simulink library "IO"  (R2024a)
settings: Solver=VariableStepAuto  StartTime=0.0  StopTime=10.0  RelTol=1e-3
values from neighbouring files (symbols this model uses):
  ADCBits = 12.0    [IO.sldd]
  Vref = 5.0    [IO.sldd]
undefined symbols (not defined in the file or in its folder): Bridge, dt, H, raptor_xcp_function
libraries: Raptor_lib x69, Utilities x20, Cooling x1
(part 1 of 3)
settings Model: Creator=serga  LastModifiedBy=hyuga
settings ConfigComp: CovBoundaryAbsTol=1.0e-5

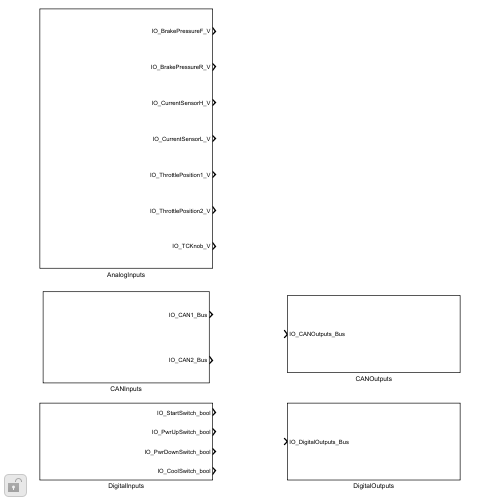
[thumbnail: Simulink's stored preview of the top-level diagram]
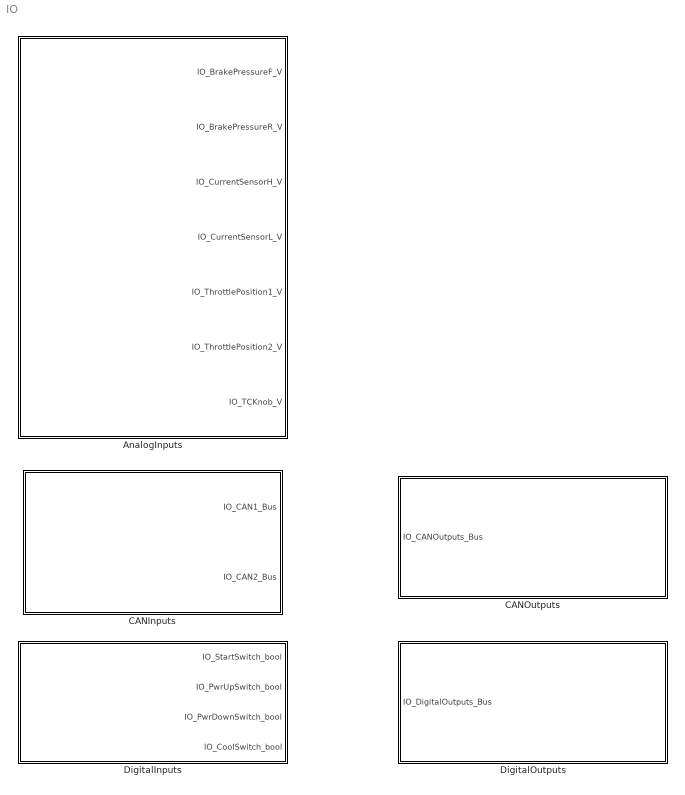
== system IO ==
  AnalogInputs : Subsystem
  CANInputs : Subsystem
  CANOutputs : Subsystem
  DigitalInputs : Subsystem
  DigitalOutputs : Subsystem

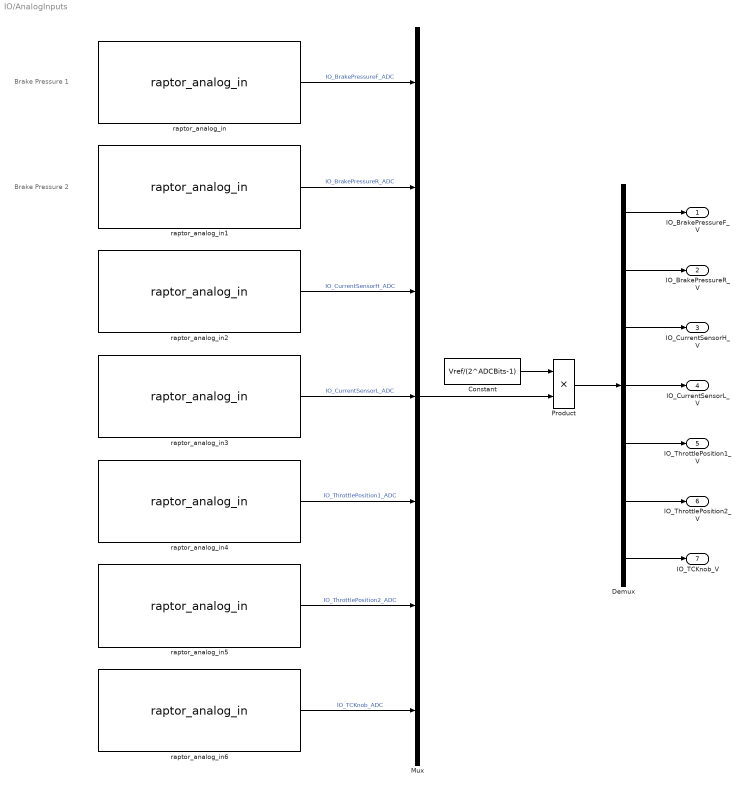
== system IO/AnalogInputs ==
  note: Brake Pressure 2
  note: Brake Pressure 1
  Constant : Constant  Value=Vref/(2^ADCBits-1)
  Demux : Demux  Outputs=7
  Mux : Mux  Inputs=7
  Product : Product
  raptor_analog_in : Raptor_lib/Input & Output/raptor_analog_in  resourceValues=INPUT2|INPUT3|INPUT4|INPUT5|INPUT6|INPUT7|INPUT8|INPUT9|INPUT10|INPUT11|INPUT12|INPUT13|INPUT14|INPUT15|INPUT16|INPUT17|INPUT18|INPUT19|INPUT20|INPUT21|INPUT22|INPUT23|INPUT24|INPUT25|INPUT26|INPUT27|INPUT28|INPUT29|INPUT30|INPUT31|INPUT32|(None)  resource=INPUT4  rangeValues=0 - 5 V  range=0 - 5 V  filterrateValues=[]  filterrate='RAPTOR MASK DEFAULT'  resolutionValues=[]  resolution=[]  pullUDValues=422k PD  pullUD=422k PD
      settings: SourceProductName=Raptor
  raptor_analog_in1 : Raptor_lib/Input & Output/raptor_analog_in  resourceValues=INPUT2|INPUT3|INPUT4|INPUT5|INPUT6|INPUT7|INPUT8|INPUT9|INPUT10|INPUT11|INPUT12|INPUT13|INPUT14|INPUT15|INPUT16|INPUT17|INPUT18|INPUT19|INPUT20|INPUT21|INPUT22|INPUT23|INPUT24|INPUT25|INPUT26|INPUT27|INPUT28|INPUT29|INPUT30|INPUT31|INPUT32|(None)  resource=INPUT12  rangeValues=0 - 5 V  range=0 - 5 V  filterrateValues=[]  filterrate='RAPTOR MASK DEFAULT'  resolutionValues=[]  resolution=[]  pullUDValues=422k PD  pullUD=422k PD
      settings: SourceProductName=Raptor
  raptor_analog_in2 : Raptor_lib/Input & Output/raptor_analog_in  resourceValues=INPUT2|INPUT3|INPUT4|INPUT5|INPUT6|INPUT7|INPUT8|INPUT9|INPUT10|INPUT11|INPUT12|INPUT13|INPUT14|INPUT15|INPUT16|INPUT17|INPUT18|INPUT19|INPUT20|INPUT21|INPUT22|INPUT23|INPUT24|INPUT25|INPUT26|INPUT27|INPUT28|INPUT29|INPUT30|INPUT31|INPUT32|(None)  resource=INPUT13  rangeValues=0 - 5 V  range=0 - 5 V  filterrateValues=[]  filterrate='RAPTOR MASK DEFAULT'  resolutionValues=[]  resolution=[]  pullUDValues=2.15k PU, 31.6k PD  pullUD=2.15k PU, 31.6k PD
      settings: SourceProductName=Raptor
  raptor_analog_in3 : Raptor_lib/Input & Output/raptor_analog_in  resourceValues=INPUT2|INPUT3|INPUT4|INPUT5|INPUT6|INPUT7|INPUT8|INPUT9|INPUT10|INPUT11|INPUT12|INPUT13|INPUT14|INPUT15|INPUT16|INPUT17|INPUT18|INPUT19|INPUT20|INPUT21|INPUT22|INPUT23|INPUT24|INPUT25|INPUT26|INPUT27|INPUT28|INPUT29|INPUT30|INPUT31|INPUT32|(None)  resource=INPUT15  rangeValues=0 - 5 V  range=0 - 5 V  filterrateValues=[]  filterrate='RAPTOR MASK DEFAULT'  resolutionValues=[]  resolution=[]  pullUDValues=2.15k PU, 31.6k PD  pullUD=2.15k PU, 31.6k PD
      settings: SourceProductName=Raptor
  raptor_analog_in4 : Raptor_lib/Input & Output/raptor_analog_in  resourceValues=INPUT2|INPUT3|INPUT4|INPUT5|INPUT6|INPUT7|INPUT8|INPUT9|INPUT10|INPUT11|INPUT12|INPUT13|INPUT14|INPUT15|INPUT16|INPUT17|INPUT18|INPUT19|INPUT20|INPUT21|INPUT22|INPUT23|INPUT24|INPUT25|INPUT26|INPUT27|INPUT28|INPUT29|INPUT30|INPUT31|INPUT32|(None)  resource=INPUT23  rangeValues=0 - 5 V  range=0 - 5 V  filterrateValues=[]  filterrate='RAPTOR MASK DEFAULT'  resolutionValues=[]  resolution=[]  pullUDValues=56.7k PD  pullUD=56.7k PD
      settings: SourceProductName=Raptor
  raptor_analog_in5 : Raptor_lib/Input & Output/raptor_analog_in  resourceValues=INPUT2|INPUT3|INPUT4|INPUT5|INPUT6|INPUT7|INPUT8|INPUT9|INPUT10|INPUT11|INPUT12|INPUT13|INPUT14|INPUT15|INPUT16|INPUT17|INPUT18|INPUT19|INPUT20|INPUT21|INPUT22|INPUT23|INPUT24|INPUT25|INPUT26|INPUT27|INPUT28|INPUT29|INPUT30|INPUT31|INPUT32|(None)  resource=INPUT24  rangeValues=0 - 5 V  range=0 - 5 V  filterrateValues=[]  filterrate='RAPTOR MASK DEFAULT'  resolutionValues=[]  resolution=[]  pullUDValues=56.7k PD  pullUD=56.7k PD
      settings: SourceProductName=Raptor
  raptor_analog_in6 : Raptor_lib/Input & Output/raptor_analog_in  resourceValues=INPUT2|INPUT3|INPUT4|INPUT5|INPUT6|INPUT7|INPUT8|INPUT9|INPUT10|INPUT11|INPUT12|INPUT13|INPUT14|INPUT15|INPUT16|INPUT17|INPUT18|INPUT19|INPUT20|INPUT21|INPUT22|INPUT23|INPUT24|INPUT25|INPUT26|INPUT27|INPUT28|INPUT29|INPUT30|INPUT31|INPUT32|(None)  resource=INPUT29  rangeValues=0 - 5 V  range=0 - 5 V  filterrateValues=[]  filterrate='RAPTOR MASK DEFAULT'  resolutionValues=[]  resolution=[]  pullUDValues=215k PD  pullUD=215k PD
      settings: SourceProductName=Raptor
  IO_BrakePressureF_V : Outport
  IO_BrakePressureR_V : Outport  Port=2
  IO_CurrentSensorH_V : Outport  Port=3
  IO_CurrentSensorL_V : Outport  Port=4
  IO_ThrottlePosition1_V : Outport  Port=5
  IO_ThrottlePosition2_V : Outport  Port=6
  IO_TCKnob_V : Outport  Port=7
  wires:
  Demux/7 -> IO_TCKnob_V/1
  Demux/6 -> IO_ThrottlePosition2_V/1
  Demux/5 -> IO_ThrottlePosition1_V/1
  Demux/4 -> IO_CurrentSensorL_V/1
  Demux/3 -> IO_CurrentSensorH_V/1
  Demux/2 -> IO_BrakePressureR_V/1
  Demux/1 -> IO_BrakePressureF_V/1
  raptor_analog_in6/1 -> Mux/7  "IO_TCKnob_ADC"
  raptor_analog_in5/1 -> Mux/6  "IO_ThrottlePosition2_ADC"
  raptor_analog_in4/1 -> Mux/5  "IO_ThrottlePosition1_ADC"
  raptor_analog_in3/1 -> Mux/4  "IO_CurrentSensorL_ADC"
  raptor_analog_in2/1 -> Mux/3  "IO_CurrentSensorH_ADC"
  raptor_analog_in1/1 -> Mux/2  "IO_BrakePressureR_ADC"
  raptor_analog_in/1 -> Mux/1  "IO_BrakePressureF_ADC"
  Product/1 -> Demux/1
  Constant/1 -> Product/1
  Mux/1 -> Product/2

== system IO/CANInputs ==
  CAN1 : Subsystem
  CAN2 : Subsystem
  IO_CAN1_Bus : Outport
  IO_CAN2_Bus : Outport  Port=2
  wires:
  CAN2/1(IO_CAN2_Bus) -> IO_CAN2_Bus/1
  CAN1/1(Out1) -> IO_CAN1_Bus/1

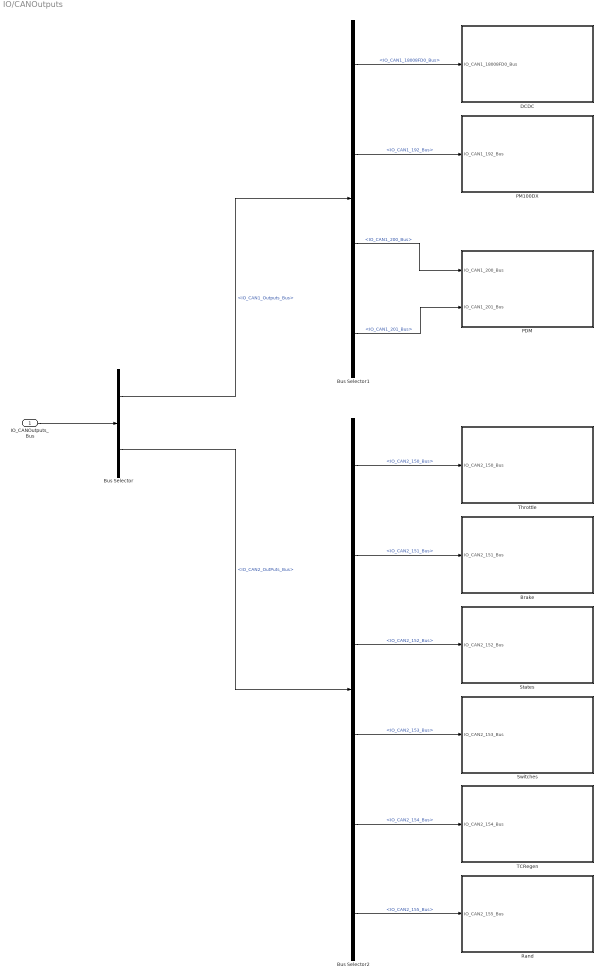
== system IO/CANOutputs ==
  IO_CANOutputs_Bus : Inport
  Brake : Subsystem
  Bus Selector : BusSelector  OutputSignals=IO_CAN1_Outputs_Bus,IO_CAN2_OutPuts_Bus
  Bus Selector1 : BusSelector  OutputSignals=IO_CAN1_18008FD0_Bus,IO_CAN1_192_Bus,IO_CAN1_200_Bus,IO_CAN1_201_Bus
  Bus Selector2 : BusSelector  OutputSignals=IO_CAN2_150_Bus,IO_CAN2_151_Bus,IO_CAN2_152_Bus,IO_CAN2_153_Bus,IO_CAN2_154_Bus,IO_CAN2_155_Bus
  DCDC : Subsystem
  PDM : Subsystem
  PM100DX : Subsystem
  Rand : Subsystem
  States : Subsystem
  Switches : Subsystem
  TCRegen : Subsystem
  Throttle : Subsystem
  wires:
  Bus Selector/2 -> Bus Selector2/1  "<IO_CAN2_OutPuts_Bus>"
  Bus Selector/1 -> Bus Selector1/1  "<IO_CAN1_Outputs_Bus>"
  IO_CANOutputs_Bus/1 -> Bus Selector/1
  Bus Selector1/1 -> DCDC/1(IO_CAN1_18008FD0_Bus)  "<IO_CAN1_18008FD0_Bus>"
  Bus Selector1/2 -> PM100DX/1(IO_CAN1_192_Bus)  "<IO_CAN1_192_Bus>"
  Bus Selector1/3 -> PDM/1(IO_CAN1_200_Bus)  "<IO_CAN1_200_Bus>"
  Bus Selector2/1 -> Throttle/1(IO_CAN2_150_Bus)  "<IO_CAN2_150_Bus>"
  Bus Selector2/2 -> Brake/1(IO_CAN2_151_Bus)  "<IO_CAN2_151_Bus>"
  Bus Selector2/3 -> States/1(IO_CAN2_152_Bus)  "<IO_CAN2_152_Bus>"
  Bus Selector2/4 -> Switches/1(IO_CAN2_153_Bus)  "<IO_CAN2_153_Bus>"
  Bus Selector1/4 -> PDM/2(IO_CAN1_201_Bus)  "<IO_CAN1_201_Bus>"
  Bus Selector2/5 -> TCRegen/1(IO_CAN2_154_Bus)  "<IO_CAN2_154_Bus>"
  Bus Selector2/6 -> Rand/1(IO_CAN2_155_Bus)  "<IO_CAN2_155_Bus>"

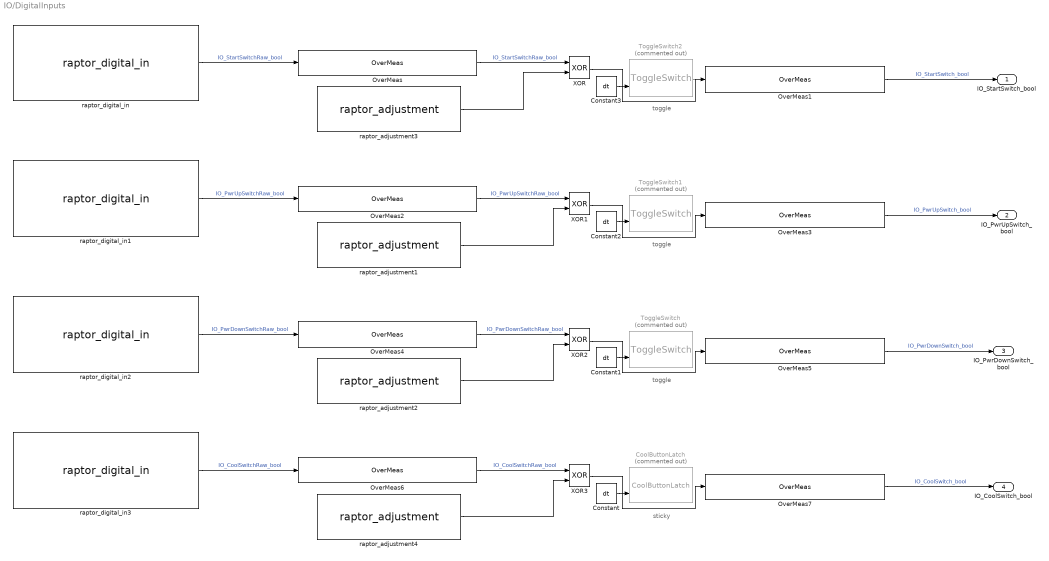
== system IO/DigitalInputs ==
  note: toggle
  note: toggle
  note: sticky
  note: toggle
  Constant{,1..3} (4 alike) : Constant  Value=dt
  CoolButtonLatch : Cooling/CoolButtonLatch  Commented=on  SystemSampleTime=-1  VariantActivationTime=update diagram  EmptyChoice=off  PassThrough=off  PassThroughVariantControl=(default)  EmptyChoiceVariantControl=(default)  AllowFlexibleInterface=on  Latency=0  AutoFrameSizeCalculation=off
  OverMeas : Utilities/OverMeas  sigName='IO_StartSwitchRaw_bool'  minimum=0  maximum=1
  OverMeas1 : Utilities/OverMeas  sigName='IO_StartSwitch_bool'  minimum=0  maximum=1
  OverMeas2 : Utilities/OverMeas  sigName='IO_PwrUpSwitchRaw_bool'  minimum=0  maximum=1
  OverMeas3 : Utilities/OverMeas  sigName='IO_PwrUpSwitch_bool'  minimum=0  maximum=1
  OverMeas4 : Utilities/OverMeas  sigName='IO_PwrDownSwitchRaw_bool'  minimum=0  maximum=1
  OverMeas5 : Utilities/OverMeas  sigName='IO_PwrDownSwitch_bool'  minimum=0  maximum=1
  OverMeas6 : Utilities/OverMeas  sigName='IO_CoolSwitchRaw_bool'  minimum=0  maximum=1
  OverMeas7 : Utilities/OverMeas  sigName='IO_CoolSwitch_bool'  minimum=0  maximum=1
  ToggleSwitch : Utilities/ToggleSwitch  Commented=on  SystemSampleTime=-1  VariantActivationTime=update diagram  EmptyChoice=off  PassThrough=off  PassThroughVariantControl=(default)  EmptyChoiceVariantControl=(default)  AllowFlexibleInterface=on  Latency=0  AutoFrameSizeCalculation=off
  ToggleSwitch1 : Utilities/ToggleSwitch  Commented=on  SystemSampleTime=-1  VariantActivationTime=update diagram  EmptyChoice=off  PassThrough=off  PassThroughVariantControl=(default)  EmptyChoiceVariantControl=(default)  AllowFlexibleInterface=on  Latency=0  AutoFrameSizeCalculation=off
  ToggleSwitch2 : Utilities/ToggleSwitch  Commented=on  SystemSampleTime=-1  VariantActivationTime=update diagram  EmptyChoice=off  PassThrough=off  PassThroughVariantControl=(default)  EmptyChoiceVariantControl=(default)  AllowFlexibleInterface=on  Latency=0  AutoFrameSizeCalculation=off
  XOR{,1..3} (4 alike) : Logic  Operator=XOR  AllPortsSameDT=off  OutDataTypeStr=boolean
  raptor_adjustment1 : Raptor_lib/Data Storage/raptor_adjustment  paramName='IO_PwrUpSwitchPolarity_bool'  nameSource=Parameter  initValue=1  dataType=uint8  storage=Calibration  calDispType=Number  calEnum={'False', 'True'}  calGain=1.0  calOffset=0.0  calMax=inf  calMin=-inf  calFormat='-1'  calUnit=''  calHelp=''  calAccess=1  calFunction=raptor_xcp_function(gcb)  calDispHeaders=off  calColHeaders={'Col1' 'Col2' 'Col3'}  calRowHeaders={'Row1' 'Row2' 'Row3'}
      settings: SourceProductName=Raptor
  raptor_adjustment2 : Raptor_lib/Data Storage/raptor_adjustment  paramName='IO_PwrDownSwitchPolarity_bool'  nameSource=Parameter  initValue=1  dataType=uint8  storage=Calibration  calDispType=Number  calEnum={'False', 'True'}  calGain=1.0  calOffset=0.0  calMax=inf  calMin=-inf  calFormat='-1'  calUnit=''  calHelp=''  calAccess=1  calFunction=raptor_xcp_function(gcb)  calDispHeaders=off  calColHeaders={'Col1' 'Col2' 'Col3'}  calRowHeaders={'Row1' 'Row2' 'Row3'}
      settings: SourceProductName=Raptor
  raptor_adjustment3 : Raptor_lib/Data Storage/raptor_adjustment  paramName='IO_StartSwitchPolarity_bool'  nameSource=Parameter  initValue=0.00  dataType=uint8  storage=Calibration  calDispType=Number  calEnum={'False', 'True'}  calGain=1.0  calOffset=0.0  calMax=inf  calMin=-inf  calFormat='-1'  calUnit=''  calHelp=''  calAccess=1  calFunction=raptor_xcp_function(gcb)  calDispHeaders=off  calColHeaders={'Col1' 'Col2' 'Col3'}  calRowHeaders={'Row1' 'Row2' 'Row3'}
      settings: SourceProductName=Raptor
  raptor_adjustment4 : Raptor_lib/Data Storage/raptor_adjustment  paramName='IO_CoolSwitchPolarity_bool'  nameSource=Parameter  initValue=1  dataType=uint8  storage=Calibration  calDispType=Number  calEnum={'False', 'True'}  calGain=1.0  calOffset=0.0  calMax=inf  calMin=-inf  calFormat='-1'  calUnit=''  calHelp=''  calAccess=1  calFunction=raptor_xcp_function(gcb)  calDispHeaders=off  calColHeaders={'Col1' 'Col2' 'Col3'}  calRowHeaders={'Row1' 'Row2' 'Row3'}
      settings: SourceProductName=Raptor
  raptor_digital_in : Raptor_lib/Input & Output/raptor_digital_in  resourceValues=WAKE_INPUT1|INPUT33|INPUT34|INPUT35|INPUT36|INPUT37|INPUT38|INPUT39|INPUT40|(None)  resource=INPUT35  pullUDValues=1.3k PD  pullUD=1.3k PD  upperThres='RAPTOR MASK DEFAULT'  lowerThres='RAPTOR MASK DEFAULT'
      settings: SourceProductName=Raptor
  raptor_digital_in1 : Raptor_lib/Input & Output/raptor_digital_in  resourceValues=WAKE_INPUT1|INPUT33|INPUT34|INPUT35|INPUT36|INPUT37|INPUT38|INPUT39|INPUT40|(None)  resource=INPUT37  pullUDValues=1.3k PU  pullUD=1.3k PU  upperThres='RAPTOR MASK DEFAULT'  lowerThres='RAPTOR MASK DEFAULT'
      settings: SourceProductName=Raptor
  raptor_digital_in2 : Raptor_lib/Input & Output/raptor_digital_in  resourceValues=WAKE_INPUT1|INPUT33|INPUT34|INPUT35|INPUT36|INPUT37|INPUT38|INPUT39|INPUT40|(None)  resource=INPUT39  pullUDValues=1.3k PU  pullUD=1.3k PU  upperThres='RAPTOR MASK DEFAULT'  lowerThres='RAPTOR MASK DEFAULT'
      settings: SourceProductName=Raptor
  raptor_digital_in3 : Raptor_lib/Input & Output/raptor_digital_in  resourceValues=WAKE_INPUT1|INPUT33|INPUT34|INPUT35|INPUT36|INPUT37|INPUT38|INPUT39|INPUT40|(None)  resource=INPUT40  pullUDValues=1.3k PU  pullUD=1.3k PU  upperThres='RAPTOR MASK DEFAULT'  lowerThres='RAPTOR MASK DEFAULT'
      settings: SourceProductName=Raptor
  IO_StartSwitch_bool : Outport
  IO_PwrUpSwitch_bool : Outport  Port=2
  IO_PwrDownSwitch_bool : Outport  Port=3
  IO_CoolSwitch_bool : Outport  Port=4
  wires:
  ToggleSwitch2/1 -> ?
  XOR/1 -> OverMeas1/1
  Constant3/1 -> ToggleSwitch2/2
  Constant2/1 -> ToggleSwitch1/2
  Constant1/1 -> ToggleSwitch/2
  Constant/1 -> CoolButtonLatch/2
  raptor_digital_in/1 -> OverMeas/1  "IO_StartSwitchRaw_bool"
  raptor_digital_in1/1 -> OverMeas2/1  "IO_PwrUpSwitchRaw_bool"
  raptor_digital_in2/1 -> OverMeas4/1  "IO_PwrDownSwitchRaw_bool"
  raptor_digital_in3/1 -> OverMeas6/1  "IO_CoolSwitchRaw_bool"
  raptor_adjustment3/1 -> XOR/2
  OverMeas/1 -> XOR/1  "IO_StartSwitchRaw_bool"
  OverMeas1/1 -> IO_StartSwitch_bool/1  "IO_StartSwitch_bool"
  OverMeas2/1 -> XOR1/1  "IO_PwrUpSwitchRaw_bool"
  OverMeas3/1 -> IO_PwrUpSwitch_bool/1  "IO_PwrUpSwitch_bool"
  raptor_adjustment1/1 -> XOR1/2
  raptor_adjustment2/1 -> XOR2/2
  OverMeas4/1 -> XOR2/1  "IO_PwrDownSwitchRaw_bool"
  OverMeas5/1 -> IO_PwrDownSwitch_bool/1  "IO_PwrDownSwitch_bool"
  OverMeas6/1 -> XOR3/1  "IO_CoolSwitchRaw_bool"
  raptor_adjustment4/1 -> XOR3/2
  OverMeas7/1 -> IO_CoolSwitch_bool/1  "IO_CoolSwitch_bool"
  XOR2/1 -> OverMeas5/1
  XOR1/1 -> OverMeas3/1
  XOR3/1 -> OverMeas7/1

== system IO/DigitalOutputs ==
  IO_DigitalOutputs_Bus : Inport
  Bus Selector1 : BusSelector  OutputSignals=IO_RTMSound_bool
  Ground : Ground
  raptor_adjustment : Raptor_lib/Data Storage/raptor_adjustment  paramName='IO_RTMSoundDuty_pct'  nameSource=Parameter  initValue=5000  dataType=int16  storage=Calibration  calDispType=Number  calEnum={'False', 'True'}  calGain=1.0  calOffset=0.0  calMax=inf  calMin=-inf  calFormat='-1'  calUnit=''  calHelp=''  calAccess=1  calFunction=raptor_xcp_function(gcb)  calDispHeaders=off  calColHeaders={'Col1' 'Col2' 'Col3'}  calRowHeaders={'Row1' 'Row2' 'Row3'}
      settings: SourceProductName=Raptor
  raptor_adjustment1 : Raptor_lib/Data Storage/raptor_adjustment  paramName='IO_RTMSoundFreq_Hz'  nameSource=Parameter  initValue=320000  dataType=uint32  storage=Calibration  calDispType=Number  calEnum={'False', 'True'}  calGain=1.0  calOffset=0.0  calMax=inf  calMin=0  calFormat='-1'  calUnit=''  calHelp=''  calAccess=1  calFunction=raptor_xcp_function(gcb)  calDispHeaders=off  calColHeaders={'Col1' 'Col2' 'Col3'}  calRowHeaders={'Row1' 'Row2' 'Row3'}
      settings: SourceProductName=Raptor
  raptor_hbridge_out : Raptor_lib/Input & Output/raptor_hbridge_out  resourceValues=OUTPUT50_51|OUTPUT52_53|OUTPUT54_55|(None)  resource=OUTPUT50_51  outError=0  driverTypeValues=H-Bridge  driverType=H-Bridge
      settings: SourceProductName=Raptor
  wires:
  IO_DigitalOutputs_Bus/1 -> Bus Selector1/1
  Bus Selector1/1 -> raptor_hbridge_out/1  "<IO_RTMSound_bool>"
  Ground/1 -> raptor_hbridge_out/2
  raptor_adjustment/1 -> raptor_hbridge_out/3
  raptor_adjustment1/1 -> raptor_hbridge_out/4

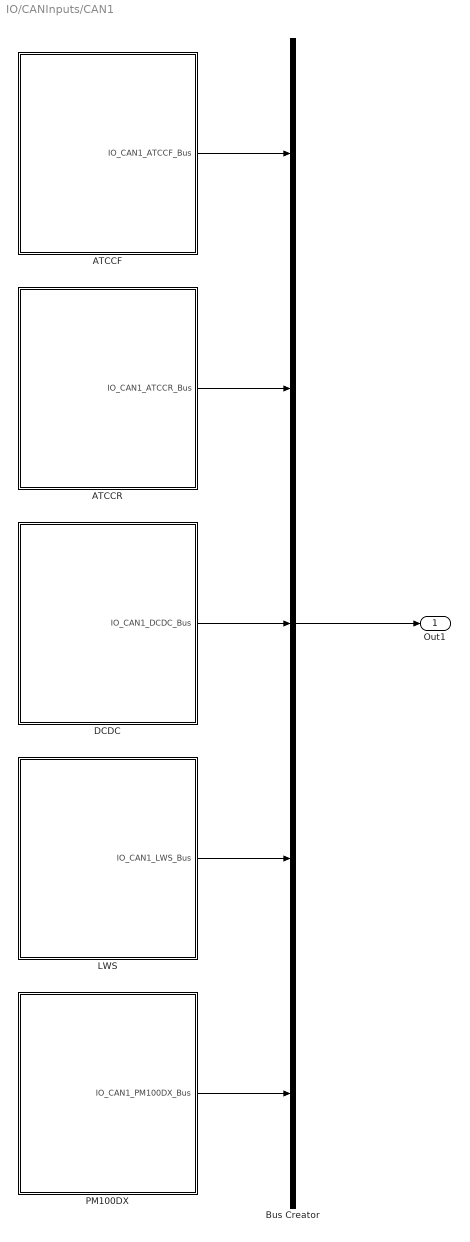
== system IO/CANInputs/CAN1 ==
  ATCCF : Subsystem
  ATCCR : Subsystem
  Bus Creator : BusCreator  Inputs=5
  DCDC : Subsystem
  LWS : Subsystem
  PM100DX : Subsystem
  Out1 : Outport
  wires:
  Bus Creator/1 -> Out1/1
  PM100DX/1(IO_CAN1_PM100DX_Bus) -> Bus Creator/5
  LWS/1(IO_CAN1_LWS_Bus) -> Bus Creator/4
  ATCCF/1(IO_CAN1_ATCCF_Bus) -> Bus Creator/1
  DCDC/1(IO_CAN1_DCDC_Bus) -> Bus Creator/3
  ATCCR/1(IO_CAN1_ATCCR_Bus) -> Bus Creator/2

== system IO/CANInputs/CAN2 ==
  BMS : Subsystem
  Bus Creator : BusCreator  Inputs=2
  MM5 : Subsystem
  IO_CAN2_Bus : Outport
  wires:
  MM5/1(IO_CAN2_MM5_Bus) -> Bus Creator/2
  BMS/1(IO_CAN2_BMS_Bus) -> Bus Creator/1
  Bus Creator/1 -> IO_CAN2_Bus/1

== system IO/CANOutputs/Brake ==
  IO_CAN2_151_Bus : Inport
  Bus Selector : BusSelector  OutputSignals=IO_BrakePressureF_psi,IO_BrakePressureR_psi
  Ground : Ground
  RollingCounterGenerator : Utilities/RollingCounterGenerator
  raptor_can_txmsg : Raptor_lib/CAN/raptor_can_txmsg  canDefinition=struct('dbcFile', 'SR26_CAN2.dbc','message', 'VCU_151','comment', '','signals', {{'VCU_brakeBias','VCU_brakePressureF','VCU_brakePressureR','VCU_counterMsg151'}},'enabled', [ 1 1 1 1;],'scaled', [ 1 1 1 1;],'canBus', '''CAN2''','messageID', [ 151;],'idMask', [ 536870911;],'payloadMask', [],'payloadValue', [],'useDbcPeriod', [ 0;],'period', [ 100;],'queueSize', [ 1;],'label', [ 0;],'ver', [ 2;],'showID', [ 0;],'showRaw', [ 0;],'showRawMsg', [ 0;],'useStartVals', [ 0;],'extendedId', [ 0;],'useSimFunc', [ 0;],'sim_func_name', '''''','fill', [ 0;],'editID', [ 0;],'signalOrder', [ 1;],'signalAscDes', [ 1;],'msgLength', [ 8;])  canBus='CAN2'  queueSize=1  payloadMask=[]  payloadValue=[]  period=100  showID=0  label=0  idMask=hex2dec('1FFFFFFF')  fill=0  id=151  showRaw=0  signalOrder=1  signalInfo={{struct('Name', 'VCU_brakePressureR','StartBit', [ 48;],'SignalSize', [ 16;],'ByteOrder', 'LittleEndian','ValueType', 'SIGNED','Class', 'int16','Signed', [ 1;],'Factor', [ 0.1;],'Offset', [ 0;],'Min', [ 0;],'Max', [ 2000;],'Units', 'psi','StartVal', [ 0;],'Comment', 'Rear brake pressure','Multiplexed', [ 0;],'Multiplexor', [ 0;],'MultiplexMode_Min', [],'MultiplexMode_Max', []),struct('Name', 'VCU_brakePressureF','StartBit', [ 32;],'SignalSize', [ 16;],'ByteOrder', 'LittleEndian','ValueType', 'SIGNED','Class', 'int16','Signed', [ 1;],'Factor', [ 0.1;],'Offset', [ 0;],'Min', [ 0;],'Max', [ 2000;],'Units', 'psi','StartVal', [ 0;],'Comment', 'Front brake pressure','Multiplexed', [ 0;],'Multiplexor', [ 0;],'MultiplexMode_Min', [],'MultiplexMode_Max', []),struct('Name', 'VCU_brakeBias','StartBit', [ 16;],'SignalSize', [ 16;],'ByteOrder', 'LittleEndian','ValueType', 'SIGNED','Class', 'int16','Signed', [ 1;],'Factor', [ 0.1;],'Offset', [ 0;],'Min', [ -3276.8;],'Max', [ 3276.7;],'Units', '%','StartVal', [ 0;],'Comment', 'Brake bias','Multiplexed', [ 0;],'Multiplexor', [ 0;],'MultiplexMode_Min', [],'MultiplexMode_Max', []),struct('Name', 'VCU_counterMsg151','StartBit', [ 0;],'SignalSize', [ 4;],'ByteOrder', 'LittleEndian','ValueType', 'UNSIGNED','Class', 'uint8','Signed', [ 0;],'Factor', [ 1;],'Offset', [ 0;],'Min', [ 0;],'Max', [ 15;],'Units', '','StartVal', [ 0;],'Comment', 'Counter Message 151','Multiplexed', [ 0;],'Multiplexor', [ 0;],'MultiplexMode_Min', [],'MultiplexMode_Max', [])}}  useSimFunc=0  sim_func_name=''  useStartVals=0
      settings: SourceProductName=Raptor
  raptor_function_call_collector : Raptor_lib/Triggers/raptor_function_call_collector  count=10
      settings: SourceProductName=Raptor
  wires:
  Ground/1 -> raptor_can_txmsg/1
  IO_CAN2_151_Bus/1 -> Bus Selector/1
  Bus Selector/1 -> raptor_can_txmsg/2  "<IO_BrakePressureF_psi>"
  Bus Selector/2 -> raptor_can_txmsg/3  "<IO_BrakePressureR_psi>"
  RollingCounterGenerator/1 -> raptor_can_txmsg/4
  raptor_function_call_collector/1 -> RollingCounterGenerator/Trigger

== system IO/CANOutputs/DCDC ==
  IO_CAN1_18008FD0_Bus : Inport
  Bus Selector : BusSelector  OutputSignals=IO_DCDCEnable_bool
  Ground : Ground
  raptor_can_txmsg : Raptor_lib/CAN/raptor_can_txmsg  canDefinition=struct('dbcFile', 'SR26_CAN1.dbc','message', 'VCU_18008FD0','comment', '','signals', {{'VCU_dcdcEnable','VCU_dcdcProtect'}},'enabled', [ 1 1;],'scaled', [ 1 1;],'canBus', '''CAN1''','messageID', [ 402690000;],'idMask', [ 536870911;],'payloadMask', [],'payloadValue', [],'useDbcPeriod', [ 0;],'period', [ 100;],'queueSize', [ 1;],'label', [ 0;],'ver', [ 2;],'showID', [ 0;],'showRaw', [ 0;],'showRawMsg', [ 0;],'useStartVals', [ 0;],'extendedId', [ 0;],'useSimFunc', [ 0;],'sim_func_name', '''''','fill', [ 0;],'editID', [ 0;],'signalOrder', [ 1;],'signalAscDes', [ 1;],'msgLength', [ 8;])  canBus='CAN1'  queueSize=1  payloadMask=[]  payloadValue=[]  period=100  showID=0  label=0  idMask=hex2dec('1FFFFFFF')  fill=0  id=402690000  showRaw=0  signalOrder=1  signalInfo={{struct('Name', 'VCU_dcdcProtect','StartBit', [ 2;],'SignalSize', [ 2;],'ByteOrder', 'LittleEndian','ValueType', 'UNSIGNED','Class', 'uint8','Signed', [ 0;],'Factor', [ 1;],'Offset', [ 0;],'Min', [ 0;],'Max', [ 0;],'Units', '','StartVal', [ 0;],'Comment', 'Protect command - once commanded, converter won`t work until restart (decimal); 1: protection confirmed','Multiplexed', [ 0;],'Multiplexor', [ 0;],'MultiplexMode_Min', [],'MultiplexMode_Max', []),struct('Name', 'VCU_dcdcEnable','StartBit', [ 0;],'SignalSize', [ 2;],'ByteOrder', 'LittleEndian','ValueType', 'UNSIGNED','Class', 'uint8','Signed', [ 0;],'Factor', [ 1;],'Offset', [ 0;],'Min', [ 0;],'Max', [ 0;],'Units', '','StartVal', [ 0;],'Comment', 'Enable command (decimal); 1: enable, 2: disable','Multiplexed', [ 0;],'Multiplexor', [ 0;],'MultiplexMode_Min', [],'MultiplexMode_Max', [])}}  useSimFunc=0  sim_func_name=''  useStartVals=0
      settings: SourceProductName=Raptor
  wires:
  IO_CAN1_18008FD0_Bus/1 -> Bus Selector/1
  Bus Selector/1 -> raptor_can_txmsg/1  "<IO_DCDCEnable_bool>"
  Ground/1 -> raptor_can_txmsg/2

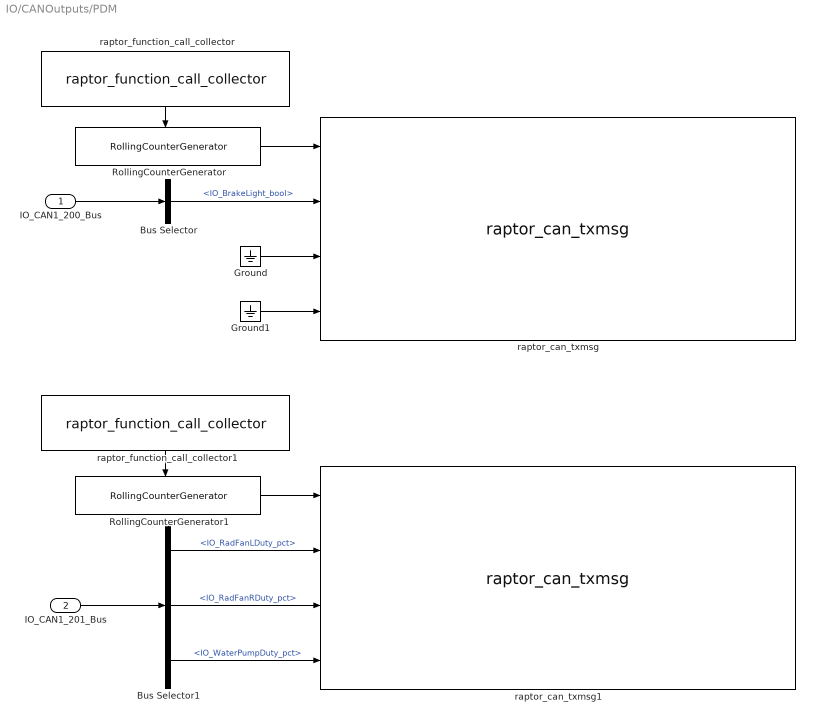
== system IO/CANOutputs/PDM ==
  IO_CAN1_200_Bus : Inport
  IO_CAN1_201_Bus : Inport  Port=2
  Bus Selector : BusSelector  OutputSignals=IO_BrakeLight_bool
  Bus Selector1 : BusSelector  OutputSignals=IO_RadFanLDuty_pct,IO_RadFanRDuty_pct,IO_WaterPumpDuty_pct
  Ground : Ground
  Ground1 : Ground
  RollingCounterGenerator : Utilities/RollingCounterGenerator
  RollingCounterGenerator1 : Utilities/RollingCounterGenerator
  raptor_can_txmsg : Raptor_lib/CAN/raptor_can_txmsg  canDefinition=struct('dbcFile', 'SR26_CAN1.dbc','message', 'VCU_200','comment', '','signals', {{'VCU_counterMsg200','VCU_brakeLightCmd','VCU_segmentHalf1Duty','VCU_segmentHalf2Duty'}},'enabled', [ 1 1 1 1;],'scaled', [ 1 1 1 1;],'canBus', '''CAN1''','messageID', [ 200;],'idMask', [ 536870911;],'payloadMask', [],'payloadValue', [],'useDbcPeriod', [ 0;],'period', [ 100;],'queueSize', [ 1;],'label', [ 0;],'ver', [ 2;],'showID', [ 0;],'showRaw', [ 0;],'showRawMsg', [ 0;],'useStartVals', [ 0;],'extendedId', [ 0;],'useSimFunc', [ 0;],'sim_func_name', '''''','fill', [ 0;],'editID', [ 0;],'signalOrder', [ 2;],'signalAscDes', [ 2;],'msgLength', [ 8;])  canBus='CAN1'  queueSize=1  payloadMask=[]  payloadValue=[]  period=100  showID=0  label=0  idMask=hex2dec('1FFFFFFF')  fill=0  id=200  showRaw=0  signalOrder=2  signalInfo={{struct('Name', 'VCU_counterMsg200','StartBit', [ 0;],'SignalSize', [ 4;],'ByteOrder', 'LittleEndian','ValueType', 'UNSIGNED','Class', 'uint8','Signed', [ 0;],'Factor', [ 1;],'Offset', [ 0;],'Min', [ 0;],'Max', [ 15;],'Units', '','StartVal', [ 0;],'Comment', 'Counter Message 200','Multiplexed', [ 0;],'Multiplexor', [ 0;],'MultiplexMode_Min', [],'MultiplexMode_Max', []),struct('Name', 'VCU_brakeLightCmd','StartBit', [ 8;],'SignalSize', [ 1;],'ByteOrder', 'LittleEndian','ValueType', 'UNSIGNED','Class', 'uint8','Signed', [ 0;],'Factor', [ 1;],'Offset', [ 0;],'Min', [ 0;],'Max', [ 1;],'Units', '','StartVal', [ 0;],'Comment', 'Brake light command, 0 = Disable, 1 = Enable','Multiplexed', [ 0;],'Multiplexor', [ 0;],'MultiplexMode_Min', [],'MultiplexMode_Max', []),struct('Name', 'VCU_segmentHalf1Duty','StartBit', [ 16;],'SignalSize', [ 16;],'ByteOrder', 'LittleEndian','ValueType', 'SIGNED','Class', 'int16','Signed', [ 1;],'Factor', [ 0.1;],'Offset', [ 0;],'Min', [ 0;],'Max', [ 100;],'Units', '%','StartVal', [ 0;],'Comment', 'Segment half 1 duty','Multiplexed', [ 0;],'Multiplexor', [ 0;],'MultiplexMode_Min', [],'MultiplexMode_Max', []),struct('Name', 'VCU_segmentHalf2Duty','StartBit', [ 32;],'SignalSize', [ 16;],'ByteOrder', 'LittleEndian','ValueType', 'SIGNED','Class', 'int16','Signed', [ 1;],'Factor', [ 0.1;],'Offset', [ 0;],'Min', [ 0;],'Max', [ 100;],'Units', '%','StartVal', [ 0;],'Comment', 'Segment half 2 duty','Multiplexed', [ 0;],'Multiplexor', [ 0;],'MultiplexMode_Min', [],'MultiplexMode_Max', [])}}  useSimFunc=0  sim_func_name=''  useStartVals=0
      settings: SourceProductName=Raptor
  raptor_can_txmsg1 : Raptor_lib/CAN/raptor_can_txmsg  canDefinition=struct('dbcFile', 'SR26_CAN1.dbc','message', 'VCU_201','comment', '','signals', {{'VCU_counterMsg201','VCU_radFanLDuty','VCU_radFanRDuty','VCU_waterPumpDuty'}},'enabled', [ 1 1 1 1;],'scaled', [ 1 1 1 1;],'canBus', '''CAN1''','messageID', [ 201;],'idMask', [ 536870911;],'payloadMask', [],'payloadValue', [],'useDbcPeriod', [ 0;],'period', [ 100;],'queueSize', [ 1;],'label', [ 0;],'ver', [ 2;],'showID', [ 0;],'showRaw', [ 0;],'showRawMsg', [ 0;],'useStartVals', [ 0;],'extendedId', [ 0;],'useSimFunc', [ 0;],'sim_func_name', '''''','fill', [ 0;],'editID', [ 0;],'signalOrder', [ 1;],'signalAscDes', [ 1;],'msgLength', [ 8;])  canBus='CAN1'  queueSize=1  payloadMask=[]  payloadValue=[]  period=100  showID=0  label=0  idMask=hex2dec('1FFFFFFF')  fill=0  id=201  showRaw=0  signalOrder=1  signalInfo={{struct('Name', 'VCU_waterPumpDuty','StartBit', [ 48;],'SignalSize', [ 16;],'ByteOrder', 'LittleEndian','ValueType', 'SIGNED','Class', 'int16','Signed', [ 1;],'Factor', [ 0.1;],'Offset', [ 0;],'Min', [ 0;],'Max', [ 100;],'Units', '%','StartVal', [ 0;],'Comment', 'Water pump duty','Multiplexed', [ 0;],'Multiplexor', [ 0;],'MultiplexMode_Min', [],'MultiplexMode_Max', []),struct('Name', 'VCU_radFanRDuty','StartBit', [ 32;],'SignalSize', [ 16;],'ByteOrder', 'LittleEndian','ValueType', 'SIGNED','Class', 'int16','Signed', [ 1;],'Factor', [ 0.1;],'Offset', [ 0;],'Min', [ 0;],'Max', [ 100;],'Units', '%','StartVal', [ 0;],'Comment', 'Right radiator fan duty','Multiplexed', [ 0;],'Multiplexor', [ 0;],'MultiplexMode_Min', [],'MultiplexMode_Max', []),struct('Name', 'VCU_radFanLDuty','StartBit', [ 16;],'SignalSize', [ 16;],'ByteOrder', 'LittleEndian','ValueType', 'SIGNED','Class', 'int16','Signed', [ 1;],'Factor', [ 0.1;],'Offset', [ 0;],'Min', [ 0;],'Max', [ 100;],'Units', '%','StartVal', [ 0;],'Comment', 'Left radiator fan duty','Multiplexed', [ 0;],'Multiplexor', [ 0;],'MultiplexMode_Min', [],'MultiplexMode_Max', []),struct('Name', 'VCU_counterMsg201','StartBit', [ 0;],'SignalSize', [ 4;],'ByteOrder', 'LittleEndian','ValueType', 'UNSIGNED','Class', 'uint8','Signed', [ 0;],'Factor', [ 1;],'Offset', [ 0;],'Min', [ 0;],'Max', [ 15;],'Units', '','StartVal', [ 0;],'Comment', 'Counter Message 201','Multiplexed', [ 0;],'Multiplexor', [ 0;],'MultiplexMode_Min', [],'MultiplexMode_Max', [])}}  useSimFunc=0  sim_func_name=''  useStartVals=0
      settings: SourceProductName=Raptor
  raptor_function_call_collector : Raptor_lib/Triggers/raptor_function_call_collector  count=10
      settings: SourceProductName=Raptor
  raptor_function_call_collector1 : Raptor_lib/Triggers/raptor_function_call_collector  count=10
      settings: SourceProductName=Raptor
  wires:
  Ground1/1 -> raptor_can_txmsg/4
  Ground/1 -> raptor_can_txmsg/3
  IO_CAN1_200_Bus/1 -> Bus Selector/1
  Bus Selector/1 -> raptor_can_txmsg/2  "<IO_BrakeLight_bool>"
  RollingCounterGenerator/1 -> raptor_can_txmsg/1
  raptor_function_call_collector/1 -> RollingCounterGenerator/Trigger
  IO_CAN1_201_Bus/1 -> Bus Selector1/1
  Bus Selector1/2 -> raptor_can_txmsg1/3  "<IO_RadFanRDuty_pct>"
  Bus Selector1/3 -> raptor_can_txmsg1/4  "<IO_WaterPumpDuty_pct>"
  Bus Selector1/1 -> raptor_can_txmsg1/2  "<IO_RadFanLDuty_pct>"
  RollingCounterGenerator1/1 -> raptor_can_txmsg1/1
  raptor_function_call_collector1/1 -> RollingCounterGenerator1/Trigger

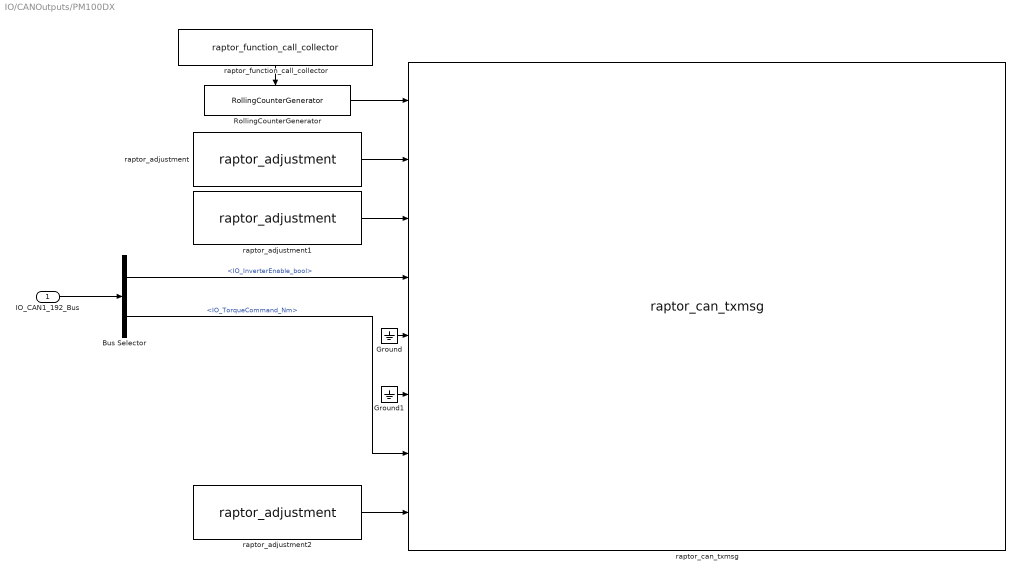
== system IO/CANOutputs/PM100DX ==
  IO_CAN1_192_Bus : Inport
  Bus Selector : BusSelector  OutputSignals=IO_InverterEnable_bool,IO_TorqueCommand_Nm
  Ground : Ground
  Ground1 : Ground
  RollingCounterGenerator : Utilities/RollingCounterGenerator
  raptor_adjustment : Raptor_lib/Data Storage/raptor_adjustment  paramName='IO_InverterDirectionCmd_bool'  nameSource=Parameter  initValue=1  dataType=boolean  storage=Calibration  calDispType=Number  calEnum={'False', 'True'}  calGain=1.0  calOffset=0.0  calMax=inf  calMin=-inf  calFormat='-1'  calUnit=''  calHelp=''  calAccess=1  calFunction=raptor_xcp_function(gcb)  calDispHeaders=off  calColHeaders={'Col1' 'Col2' 'Col3'}  calRowHeaders={'Row1' 'Row2' 'Row3'}
      settings: SourceProductName=Raptor
  raptor_adjustment1 : Raptor_lib/Data Storage/raptor_adjustment  paramName='IO_InverterDischargeCmd_bool'  nameSource=Parameter  initValue=0  dataType=boolean  storage=Calibration  calDispType=Number  calEnum={'False', 'True'}  calGain=1.0  calOffset=0.0  calMax=inf  calMin=-inf  calFormat='-1'  calUnit=''  calHelp=''  calAccess=1  calFunction=raptor_xcp_function(gcb)  calDispHeaders=off  calColHeaders={'Col1' 'Col2' 'Col3'}  calRowHeaders={'Row1' 'Row2' 'Row3'}
      settings: SourceProductName=Raptor
  raptor_adjustment2 : Raptor_lib/Data Storage/raptor_adjustment  paramName='IO_InverterTorqueLimit_Nm'  nameSource=Parameter  initValue=240  dataType=single  storage=Calibration  calDispType=Number  calEnum={'False', 'True'}  calGain=1.0  calOffset=0.0  calMax=inf  calMin=-inf  calFormat='-1'  calUnit=''  calHelp=''  calAccess=1  calFunction=raptor_xcp_function(gcb)  calDispHeaders=off  calColHeaders={'Col1' 'Col2' 'Col3'}  calRowHeaders={'Row1' 'Row2' 'Row3'}
      settings: SourceProductName=Raptor
  raptor_can_txmsg : Raptor_lib/CAN/raptor_can_txmsg  canDefinition=struct('dbcFile', 'SR26_CAN1.dbc','message', 'VCU_192','comment', '','signals', {{'VCU_counterMsg192','VCU_directionCommand','VCU_inverterDischarge','VCU_inverterEnable','VCU_speedCommand','VCU_speedModeEnable','VCU_torqueCommand','VCU_torqueLimitCommand'}},'enabled', [ 1 1 1 1 1 1 1 1;],'scaled', [ 1 1 1 1 1 1 1 1;],'canBus', '''CAN1''','messageID', [ 192;],'idMask', [ 536870911;],'payloadMask', [],'payloadValue', [],'useDbcPeriod', [ 0;],'period', [ 100;],'queueSize', [ 1;],'label', [ 0;],'ver', [ 2;],'showID', [ 0;],'showRaw', [ 0;],'showRawMsg', [ 0;],'useStartVals', [ 0;],'extendedId', [ 0;],'useSimFunc', [ 0;],'sim_func_name', '''''','fill', [ 0;],'editID', [ 0;],'signalOrder', [ 1;],'signalAscDes', [ 1;],'msgLength', [ 8;])  canBus='CAN1'  queueSize=1  payloadMask=[]  payloadValue=[]  period=100  showID=0  label=0  idMask=hex2dec('1FFFFFFF')  fill=0  id=192  showRaw=0  signalOrder=1  signalInfo={{struct('Name', 'VCU_torqueLimitCommand','StartBit', [ 48;],'SignalSize', [ 16;],'ByteOrder', 'LittleEndian','ValueType', 'SIGNED','Class', 'int16','Signed', [ 1;],'Factor', [ 0.1;],'Offset', [ 0;],'Min', [ -3276.8;],'Max', [ 3276.7;],'Units', 'Nm','StartVal', [ 0;],'Comment', 'Torque Limit - set to 0 to keep default','Multiplexed', [ 0;],'Multiplexor', [ 0;],'MultiplexMode_Min', [],'MultiplexMode_Max', []),struct('Name', 'VCU_counterMsg192','StartBit', [ 44;],'SignalSize', [ 4;],'ByteOrder', 'LittleEndian','ValueType', 'UNSIGNED','Class', 'uint8','Signed', [ 0;],'Factor', [ 1;],'Offset', [ 0;],'Min', [ 0;],'Max', [ 15;],'Units', '','StartVal', [ 0;],'Comment', 'Counter Message 192 (reserved for future use/other models)','Multiplexed', [ 0;],'Multiplexor', [ 0;],'MultiplexMode_Min', [],'MultiplexMode_Max', []),struct('Name', 'VCU_speedModeEnable','StartBit', [ 42;],'SignalSize', [ 1;],'ByteOrder', 'LittleEndian','ValueType', 'UNSIGNED','Class', 'uint8','Signed', [ 0;],'Factor', [ 1;],'Offset', [ 0;],'Min', [ 0;],'Max', [ 1;],'Units', '','StartVal', [ 0;],'Comment', '0 = No Change Mode, 1 = Change to Speed Mode from Torque Mode','Multiplexed', [ 0;],'Multiplexor', [ 0;],'MultiplexMode_Min', [],'MultiplexMode_Max', []),struct('Name', 'VCU_inverterDischarge','StartBit', [ 41;],'SignalSize', [ 1;],'ByteOrder', 'LittleEndian','ValueType', 'UNSIGNED','Class', 'uint8','Signed', [ 0;],'Factor', [ 1;],'Offset', [ 0;],'Min', [ 0;],'Max', [ 1;],'Units', '','StartVal', [ 0;],'Comment', '0 = Discharge Disable, 1 = Discharge Enable','Multiplexed', [ 0;],'Multiplexor', [ 0;],'MultiplexMode_Min', [],'MultiplexMode_Max', []),struct('Name', 'VCU_inverterEnable','StartBit', [ 40;],'SignalSize', [ 1;],'ByteOrder', 'LittleEndian','ValueType', 'UNSIGNED','Class', 'uint8','Signed', [ 0;],'Factor', [ 1;],'Offset', [ 0;],'Min', [ 0;],'Max', [ 1;],'Units', '','StartVal', [ 0;],'Comment', '0 = Inverter OFF, 1 = Inverter ON','Multiplexed', [ 0;],'Multiplexor', [ 0;],'MultiplexMode_Min', [],'MultiplexMode_Max', []),struct('Name', 'VCU_directionCommand','StartBit', [ 32;],'SignalSize', [ 1;],'ByteOrder', 'LittleEndian','ValueType', 'UNSIGNED','Class', 'uint8','Signed', [ 0;],'Factor', [ 1;],'Offset', [ 0;],'Min', [ 0;],'Max', [ 1;],'Units', '','StartVal', [ 0;],'Comment', '0 = CW, 1 = CCW, viewed from the shaft end of the motor','Multiplexed', [ 0;],'Multiplexor', [ 0;],'MultiplexMode_Min', [],'MultiplexMode_Max', []),struct('Name', 'VCU_speedCommand','StartBit', [ 16;],'SignalSize', [ 16;],'ByteOrder', 'LittleEndian','ValueType', 'SIGNED','Class', 'int16','Signed', [ 1;],'Factor', [ 1;],'Offset', [ 0;],'Min', [ -32768;],'Max', [ 32767;],'Units', 'rpm','StartVal', [ 0;],'Comment', 'Speed Command when used in Speed Mode','Multiplexed', [ 0;],'Multiplexor', [ 0;],'MultiplexMode_Min', [],'MultiplexMode_Max', []),struct('Name', 'VCU_torqueCommand','StartBit', [ 0;],'SignalSize', [ 16;],'ByteOrder', 'LittleEndian','ValueType', 'SIGNED','Class', 'int16','Signed', [ 1;],'Factor', [ 0.1;],'Offset', [ 0;],'Min', [ -3276.8;],'Max', [ 3276.7;],'Units', 'Nm','StartVal', [ 0;],'Comment', 'Torque Command in Torque Mode','Multiplexed', [ 0;],'Multiplexor', [ 0;],'MultiplexMode_Min', [],'MultiplexMode_Max', [])}}  useSimFunc=0  sim_func_name=''  useStartVals=0
      settings: SourceProductName=Raptor
  raptor_function_call_collector : Raptor_lib/Triggers/raptor_function_call_collector  count=10
      settings: SourceProductName=Raptor
  wires:
  IO_CAN1_192_Bus/1 -> Bus Selector/1
  Bus Selector/1 -> raptor_can_txmsg/4  "<IO_InverterEnable_bool>"
  Bus Selector/2 -> raptor_can_txmsg/7  "<IO_TorqueCommand_Nm>"
  Ground/1 -> raptor_can_txmsg/5
  Ground1/1 -> raptor_can_txmsg/6
  RollingCounterGenerator/1 -> raptor_can_txmsg/1
  raptor_adjustment/1 -> raptor_can_txmsg/2
  raptor_adjustment1/1 -> raptor_can_txmsg/3
  raptor_adjustment2/1 -> raptor_can_txmsg/8
  raptor_function_call_collector/1 -> RollingCounterGenerator/Trigger

== system IO/CANOutputs/Rand ==
  IO_CAN2_155_Bus : Inport
  Bus Selector : BusSelector  OutputSignals=CTRL_AssistedTorque_Nm,IO_ContactorFault_en,IO_DriveSpeed_mph
  RollingCounterGenerator : Utilities/RollingCounterGenerator
  raptor_can_txmsg : Raptor_lib/CAN/raptor_can_txmsg  canDefinition=struct('dbcFile', 'SR26_CAN2.dbc','message', 'VCU_155','comment', '','signals', {{'VCU_assistedTorque','VCU_contactorFault','VCU_counterMsg155','VCU_driveSpeed'}},'enabled', [ 1 1 1 1;],'scaled', [ 1 1 1 1;],'canBus', '''CAN2''','messageID', [ 155;],'idMask', [ 536870911;],'payloadMask', [],'payloadValue', [],'useDbcPeriod', [ 0;],'period', [ 100;],'queueSize', [ 1;],'label', [ 0;],'ver', [ 2;],'showID', [ 0;],'showRaw', [ 0;],'showRawMsg', [ 0;],'useStartVals', [ 0;],'extendedId', [ 0;],'useSimFunc', [ 0;],'sim_func_name', '''''','fill', [ 0;],'editID', [ 0;],'signalOrder', [ 1;],'signalAscDes', [ 1;],'msgLength', [ 8;])  canBus='CAN2'  queueSize=1  payloadMask=[]  payloadValue=[]  period=100  showID=0  label=0  idMask=hex2dec('1FFFFFFF')  fill=0  id=155  showRaw=0  signalOrder=1  signalInfo={{struct('Name', 'VCU_contactorFault','StartBit', [ 48;],'SignalSize', [ 8;],'ByteOrder', 'LittleEndian','ValueType', 'UNSIGNED','Class', 'uint8','Signed', [ 0;],'Factor', [ 1;],'Offset', [ 0;],'Min', [ 0;],'Max', [ 255;],'Units', '','StartVal', [ 0;],'Comment', 'Signal to fire contactors to BMS (enumerated)','Multiplexed', [ 0;],'Multiplexor', [ 0;],'MultiplexMode_Min', [],'MultiplexMode_Max', []),struct('Name', 'VCU_assistedTorque','StartBit', [ 32;],'SignalSize', [ 16;],'ByteOrder', 'LittleEndian','ValueType', 'SIGNED','Class', 'int16','Signed', [ 1;],'Factor', [ 0.1;],'Offset', [ 0;],'Min', [ -300;],'Max', [ 300;],'Units', 'Nm','StartVal', [ 0;],'Comment', 'Torque after brake regen and TC','Multiplexed', [ 0;],'Multiplexor', [ 0;],'MultiplexMode_Min', [],'MultiplexMode_Max', []),struct('Name', 'VCU_driveSpeed','StartBit', [ 16;],'SignalSize', [ 16;],'ByteOrder', 'LittleEndian','ValueType', 'SIGNED','Class', 'int16','Signed', [ 1;],'Factor', [ 0.1;],'Offset', [ 0;],'Min', [ -20;],'Max', [ 3276.7;],'Units', 'mph','StartVal', [ 0;],'Comment', 'Front wheel speed','Multiplexed', [ 0;],'Multiplexor', [ 0;],'MultiplexMode_Min', [],'MultiplexMode_Max', []),struct('Name', 'VCU_counterMsg155','StartBit', [ 0;],'SignalSize', [ 4;],'ByteOrder', 'LittleEndian','ValueType', 'UNSIGNED','Class', 'uint8','Signed', [ 0;],'Factor', [ 1;],'Offset', [ 0;],'Min', [ 0;],'Max', [ 15;],'Units', '','StartVal', [ 0;],'Comment', 'Counter Message 155','Multiplexed', [ 0;],'Multiplexor', [ 0;],'MultiplexMode_Min', [],'MultiplexMode_Max', [])}}  useSimFunc=0  sim_func_name=''  useStartVals=0
      settings: SourceProductName=Raptor
  raptor_function_call_collector : Raptor_lib/Triggers/raptor_function_call_collector  count=10
      settings: SourceProductName=Raptor
  wires:
  Bus Selector/3 -> raptor_can_txmsg/4  "<IO_DriveSpeed_mph>"
  Bus Selector/2 -> raptor_can_txmsg/2  "<IO_ContactorFault_en>"
  Bus Selector/1 -> raptor_can_txmsg/1  "<CTRL_AssistedTorque_Nm>"
  IO_CAN2_155_Bus/1 -> Bus Selector/1
  RollingCounterGenerator/1 -> raptor_can_txmsg/3
  raptor_function_call_collector/1 -> RollingCounterGenerator/Trigger

== system IO/CANOutputs/States ==
  IO_CAN2_152_Bus : Inport
  Bus Selector : BusSelector  OutputSignals=IO_RTMSound_bool,IO_TCDial_na,IO_TorqueCurve_en,IO_TorqueProfile_en,IO_VehicleState_en
  RollingCounterGenerator : Utilities/RollingCounterGenerator
  raptor_can_txmsg : Raptor_lib/CAN/raptor_can_txmsg  canDefinition=struct('dbcFile', 'SR26_CAN2.dbc','message', 'VCU_152','comment', '','signals', {{'VCU_counterMsg152','VCU_rtmSound','VCU_tCDial','VCU_torqueCurve','VCU_torqueProfile','VCU_vehicleState'}},'enabled', [ 1 1 1 1 1 1;],'scaled', [ 1 1 1 1 1 1;],'canBus', '''CAN2''','messageID', [ 152;],'idMask', [ 536870911;],'payloadMask', [],'payloadValue', [],'useDbcPeriod', [ 0;],'period', [ 100;],'queueSize', [ 1;],'label', [ 0;],'ver', [ 2;],'showID', [ 0;],'showRaw', [ 0;],'showRawMsg', [ 0;],'useStartVals', [ 0;],'extendedId', [ 0;],'useSimFunc', [ 0;],'sim_func_name', '''''','fill', [ 0;],'editID', [ 0;],'signalOrder', [ 1;],'signalAscDes', [ 1;],'msgLength', [ 8;])  canBus='CAN2'  queueSize=1  payloadMask=[]  payloadValue=[]  period=100  showID=0  label=0  idMask=hex2dec('1FFFFFFF')  fill=0  id=152  showRaw=0  signalOrder=1  signalInfo={{struct('Name', 'VCU_rtmSound','StartBit', [ 40;],'SignalSize', [ 1;],'ByteOrder', 'LittleEndian','ValueType', 'UNSIGNED','Class', 'uint8','Signed', [ 0;],'Factor', [ 1;],'Offset', [ 0;],'Min', [ 0;],'Max', [ 1;],'Units', '','StartVal', [ 0;],'Comment', 'Ready to move sound','Multiplexed', [ 0;],'Multiplexor', [ 0;],'MultiplexMode_Min', [],'MultiplexMode_Max', []),struct('Name', 'VCU_torqueCurve','StartBit', [ 32;],'SignalSize', [ 8;],'ByteOrder', 'LittleEndian','ValueType', 'UNSIGNED','Class', 'uint8','Signed', [ 0;],'Factor', [ 1;],'Offset', [ 0;],'Min', [ 0;],'Max', [ 255;],'Units', '','StartVal', [ 0;],'Comment', 'Torque curve (enumerated in DBC value table)','Multiplexed', [ 0;],'Multiplexor', [ 0;],'MultiplexMode_Min', [],'MultiplexMode_Max', []),struct('Name', 'VCU_torqueProfile','StartBit', [ 24;],'SignalSize', [ 8;],'ByteOrder', 'LittleEndian','ValueType', 'UNSIGNED','Class', 'uint8','Signed', [ 0;],'Factor', [ 1;],'Offset', [ 0;],'Min', [ 0;],'Max', [ 255;],'Units', '','StartVal', [ 0;],'Comment', 'Torque profile (enumerated in DBC value table)','Multiplexed', [ 0;],'Multiplexor', [ 0;],'MultiplexMode_Min', [],'MultiplexMode_Max', []),struct('Name', 'VCU_tCDial','StartBit', [ 16;],'SignalSize', [ 8;],'ByteOrder', 'LittleEndian','ValueType', 'UNSIGNED','Class', 'uint8','Signed', [ 0;],'Factor', [ 1;],'Offset', [ 0;],'Min', [ 0;],'Max', [ 255;],'Units', '','StartVal', [ 0;],'Comment', '','Multiplexed', [ 0;],'Multiplexor', [ 0;],'MultiplexMode_Min', [],'MultiplexMode_Max', []),struct('Name', 'VCU_vehicleState','StartBit', [ 8;],'SignalSize', [ 8;],'ByteOrder', 'LittleEndian','ValueType', 'UNSIGNED','Class', 'uint8','Signed', [ 0;],'Factor', [ 1;],'Offset', [ 0;],'Min', [ 0;],'Max', [ 255;],'Units', '','StartVal', [ 0;],'Comment', 'Vehicle state (enumerated in DBC value table)','Multiplexed', [ 0;],'Multiplexor', [ 0;],'MultiplexMode_Min', [],'MultiplexMode_Max', []),struct('Name', 'VCU_counterMsg152','StartBit', [ 0;],'SignalSize', [ 4;],'ByteOrder', 'LittleEndian','ValueType', 'UNSIGNED','Class', 'uint8','Signed', [ 0;],'Factor', [ 1;],'Offset', [ 0;],'Min', [ 0;],'Max', [ 15;],'Units', '','StartVal', [ 0;],'Comment', 'Counter Message 152','Multiplexed', [ 0;],'Multiplexor', [ 0;],'MultiplexMode_Min', [],'MultiplexMode_Max', [])}}  useSimFunc=0  sim_func_name=''  useStartVals=0
      settings: SourceProductName=Raptor
  raptor_function_call_collector : Raptor_lib/Triggers/raptor_function_call_collector  count=10
      settings: SourceProductName=Raptor
  wires:
  Bus Selector/5 -> raptor_can_txmsg/6  "<IO_VehicleState_en>"
  Bus Selector/4 -> raptor_can_txmsg/5  "<IO_TorqueProfile_en>"
  Bus Selector/3 -> raptor_can_txmsg/4  "<IO_TorqueCurve_en>"
  Bus Selector/2 -> raptor_can_txmsg/3  "<IO_TCDial_na>"
  Bus Selector/1 -> raptor_can_txmsg/2  "<IO_RTMSound_bool>"
  IO_CAN2_152_Bus/1 -> Bus Selector/1
  raptor_function_call_collector/1 -> RollingCounterGenerator/Trigger
  RollingCounterGenerator/1 -> raptor_can_txmsg/1

== system IO/CANOutputs/Switches ==
  IO_CAN2_153_Bus : Inport
  Bus Selector : BusSelector  OutputSignals=IO_CoolSwitch_bool,IO_PwrDownSwitch_bool,IO_PwrUpSwitch_bool,IO_StartSwitch_bool
  RollingCounterGenerator : Utilities/RollingCounterGenerator
  raptor_can_txmsg : Raptor_lib/CAN/raptor_can_txmsg  canDefinition=struct('dbcFile', 'SR26_CAN2.dbc','message', 'VCU_153','comment', '','signals', {{'VCU_coolSwitch','VCU_counterMsg153','VCU_pwrDownSwitch','VCU_pwrUpSwitch','VCU_startSwitch'}},'enabled', [ 1 1 1 1 1;],'scaled', [ 1 1 1 1 1;],'canBus', '''CAN2''','messageID', [ 153;],'idMask', [ 536870911;],'payloadMask', [],'payloadValue', [],'useDbcPeriod', [ 0;],'period', [ 100;],'queueSize', [ 1;],'label', [ 0;],'ver', [ 2;],'showID', [ 0;],'showRaw', [ 0;],'showRawMsg', [ 0;],'useStartVals', [ 0;],'extendedId', [ 0;],'useSimFunc', [ 0;],'sim_func_name', '''''','fill', [ 0;],'editID', [ 0;],'signalOrder', [ 1;],'signalAscDes', [ 1;],'msgLength', [ 8;])  canBus='CAN2'  queueSize=1  payloadMask=[]  payloadValue=[]  period=100  showID=0  label=0  idMask=hex2dec('1FFFFFFF')  fill=0  id=153  showRaw=0  signalOrder=1  signalInfo={{struct('Name', 'VCU_coolSwitch','StartBit', [ 32;],'SignalSize', [ 1;],'ByteOrder', 'LittleEndian','ValueType', 'UNSIGNED','Class', 'uint8','Signed', [ 0;],'Factor', [ 1;],'Offset', [ 0;],'Min', [ 0;],'Max', [ 1;],'Units', '','StartVal', [ 0;],'Comment', 'Cool switch signal','Multiplexed', [ 0;],'Multiplexor', [ 0;],'MultiplexMode_Min', [],'MultiplexMode_Max', []),struct('Name', 'VCU_pwrDownSwitch','StartBit', [ 24;],'SignalSize', [ 1;],'ByteOrder', 'LittleEndian','ValueType', 'UNSIGNED','Class', 'uint8','Signed', [ 0;],'Factor', [ 1;],'Offset', [ 0;],'Min', [ 0;],'Max', [ 1;],'Units', '','StartVal', [ 0;],'Comment', 'Power down switch signal','Multiplexed', [ 0;],'Multiplexor', [ 0;],'MultiplexMode_Min', [],'MultiplexMode_Max', []),struct('Name', 'VCU_pwrUpSwitch','StartBit', [ 16;],'SignalSize', [ 1;],'ByteOrder', 'LittleEndian','ValueType', 'UNSIGNED','Class', 'uint8','Signed', [ 0;],'Factor', [ 1;],'Offset', [ 0;],'Min', [ 0;],'Max', [ 1;],'Units', '','StartVal', [ 0;],'Comment', 'Power up switch signal','Multiplexed', [ 0;],'Multiplexor', [ 0;],'MultiplexMode_Min', [],'MultiplexMode_Max', []),struct('Name', 'VCU_startSwitch','StartBit', [ 8;],'SignalSize', [ 1;],'ByteOrder', 'LittleEndian','ValueType', 'UNSIGNED','Class', 'uint8','Signed', [ 0;],'Factor', [ 1;],'Offset', [ 0;],'Min', [ 0;],'Max', [ 1;],'Units', '','StartVal', [ 0;],'Comment', 'Start switch signal','Multiplexed', [ 0;],'Multiplexor', [ 0;],'MultiplexMode_Min', [],'MultiplexMode_Max', []),struct('Name', 'VCU_counterMsg153','StartBit', [ 0;],'SignalSize', [ 4;],'ByteOrder', 'LittleEndian','ValueType', 'UNSIGNED','Class', 'uint8','Signed', [ 0;],'Factor', [ 1;],'Offset', [ 0;],'Min', [ 0;],'Max', [ 15;],'Units', '','StartVal', [ 0;],'Comment', 'Counter Message 153','Multiplexed', [ 0;],'Multiplexor', [ 0;],'MultiplexMode_Min', [],'MultiplexMode_Max', [])}}  useSimFunc=0  sim_func_name=''  useStartVals=0
      settings: SourceProductName=Raptor
  raptor_function_call_collector : Raptor_lib/Triggers/raptor_function_call_collector  count=10
      settings: SourceProductName=Raptor
  wires:
  IO_CAN2_153_Bus/1 -> Bus Selector/1
  Bus Selector/1 -> raptor_can_txmsg/1  "<IO_CoolSwitch_bool>"
  Bus Selector/2 -> raptor_can_txmsg/3  "<IO_PwrDownSwitch_bool>"
  Bus Selector/3 -> raptor_can_txmsg/4  "<IO_PwrUpSwitch_bool>"
  Bus Selector/4 -> raptor_can_txmsg/5  "<IO_StartSwitch_bool>"
  RollingCounterGenerator/1 -> raptor_can_txmsg/2
  raptor_function_call_collector/1 -> RollingCounterGenerator/Trigger

== system IO/CANOutputs/TCRegen ==
  IO_CAN2_154_Bus : Inport
  Bus Selector : BusSelector  OutputSignals=IO_RegenEnable_en,IO_TCActive_bool,IO_TCEnable_en,IO_TCSensitivity_en
  RollingCounterGenerator : Utilities/RollingCounterGenerator
  raptor_can_txmsg : Raptor_lib/CAN/raptor_can_txmsg  canDefinition=struct('dbcFile', 'SR26_CAN2.dbc','message', 'VCU_154','comment', '','signals', {{'VCU_counterMsg154','VCU_regenEnable','VCU_tCActive','VCU_tCEnable','VCU_tCSensitivity'}},'enabled', [ 1 1 1 1 1;],'scaled', [ 1 1 1 1 1;],'canBus', '''CAN2''','messageID', [ 154;],'idMask', [ 536870911;],'payloadMask', [],'payloadValue', [],'useDbcPeriod', [ 0;],'period', [ 100;],'queueSize', [ 1;],'label', [ 0;],'ver', [ 2;],'showID', [ 0;],'showRaw', [ 0;],'showRawMsg', [ 0;],'useStartVals', [ 0;],'extendedId', [ 0;],'useSimFunc', [ 0;],'sim_func_name', '''''','fill', [ 0;],'editID', [ 0;],'signalOrder', [ 1;],'signalAscDes', [ 1;],'msgLength', [ 8;])  canBus='CAN2'  queueSize=1  payloadMask=[]  payloadValue=[]  period=100  showID=0  label=0  idMask=hex2dec('1FFFFFFF')  fill=0  id=154  showRaw=0  signalOrder=1  signalInfo={{struct('Name', 'VCU_regenEnable','StartBit', [ 48;],'SignalSize', [ 8;],'ByteOrder', 'LittleEndian','ValueType', 'UNSIGNED','Class', 'uint8','Signed', [ 0;],'Factor', [ 1;],'Offset', [ 0;],'Min', [ 0;],'Max', [ 255;],'Units', '','StartVal', [ 0;],'Comment', 'Enumeration','Multiplexed', [ 0;],'Multiplexor', [ 0;],'MultiplexMode_Min', [],'MultiplexMode_Max', []),struct('Name', 'VCU_tCEnable','StartBit', [ 40;],'SignalSize', [ 8;],'ByteOrder', 'LittleEndian','ValueType', 'UNSIGNED','Class', 'uint8','Signed', [ 0;],'Factor', [ 1;],'Offset', [ 0;],'Min', [ 0;],'Max', [ 255;],'Units', '','StartVal', [ 0;],'Comment', 'Enumeration','Multiplexed', [ 0;],'Multiplexor', [ 0;],'MultiplexMode_Min', [],'MultiplexMode_Max', []),struct('Name', 'VCU_tCActive','StartBit', [ 32;],'SignalSize', [ 8;],'ByteOrder', 'LittleEndian','ValueType', 'UNSIGNED','Class', 'uint8','Signed', [ 0;],'Factor', [ 1;],'Offset', [ 0;],'Min', [ 0;],'Max', [ 255;],'Units', '','StartVal', [ 0;],'Comment', '0 = off, 1 = on Enumeration','Multiplexed', [ 0;],'Multiplexor', [ 0;],'MultiplexMode_Min', [],'MultiplexMode_Max', []),struct('Name', 'VCU_tCSensitivity','StartBit', [ 16;],'SignalSize', [ 16;],'ByteOrder', 'LittleEndian','ValueType', 'UNSIGNED','Class', 'uint16','Signed', [ 0;],'Factor', [ 1;],'Offset', [ 0;],'Min', [ -20;],'Max', [ 3276.7;],'Units', '','StartVal', [ 0;],'Comment', '','Multiplexed', [ 0;],'Multiplexor', [ 0;],'MultiplexMode_Min', [],'MultiplexMode_Max', []),struct('Name', 'VCU_counterMsg154','StartBit', [ 0;],'SignalSize', [ 4;],'ByteOrder', 'LittleEndian','ValueType', 'UNSIGNED','Class', 'uint8','Signed', [ 0;],'Factor', [ 1;],'Offset', [ 0;],'Min', [ 0;],'Max', [ 15;],'Units', '','StartVal', [ 0;],'Comment', 'Counter Message 154','Multiplexed', [ 0;],'Multiplexor', [ 0;],'MultiplexMode_Min', [],'MultiplexMode_Max', [])}}  useSimFunc=0  sim_func_name=''  useStartVals=0
      settings: SourceProductName=Raptor
  raptor_function_call_collector : Raptor_lib/Triggers/raptor_function_call_collector  count=10
      settings: SourceProductName=Raptor
  wires:
  Bus Selector/4 -> raptor_can_txmsg/5  "<IO_TCSensitivity_en>"
  Bus Selector/3 -> raptor_can_txmsg/4  "<IO_TCEnable_en>"
  Bus Selector/2 -> raptor_can_txmsg/3  "<IO_TCActive_bool>"
  Bus Selector/1 -> raptor_can_txmsg/2  "<IO_RegenEnable_en>"
  IO_CAN2_154_Bus/1 -> Bus Selector/1
  raptor_function_call_collector/1 -> RollingCounterGenerator/Trigger
  RollingCounterGenerator/1 -> raptor_can_txmsg/1
